simulink model "heyangjiang"  (Simulink 6.0)
settings: Solver=ode45  StartTime=0.0  StopTime=10.0  RelTol=1e-3
libraries: dsparch4 x2, commchan2 x1, dspxfrm3 x1, commsynccomp2 x1
settings Model: LastModifiedBy=xxgcxy602

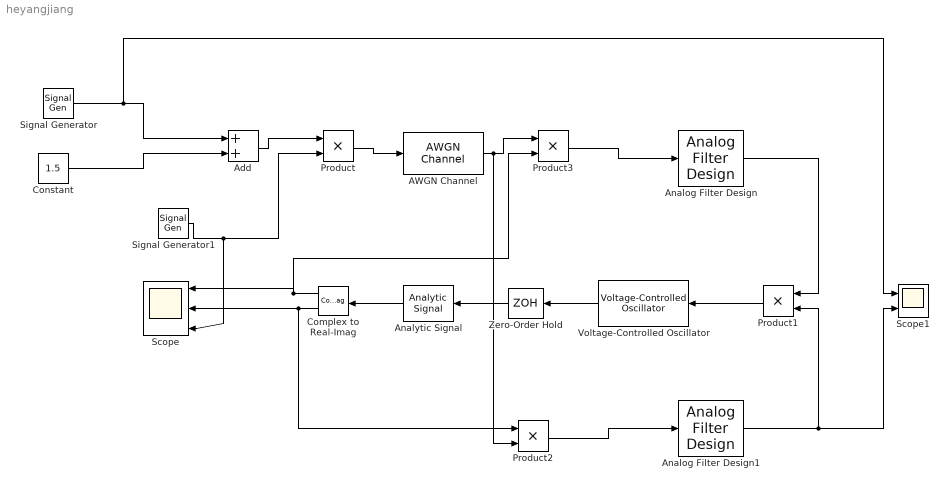
== system heyangjiang ==
  AWGN Channel : commchan2/AWGN Channel  seed=0  noiseMode=Variance from mask  EbNodB=10  EsNodB=10  SNRdB=10  bitsPerSym=1  Ps=1  Tsym=1  variance=0.01
  Add : Sum  OutScaling=2^-10
  Analog Filter Design : dsparch4/Analog Filter Design  method=Butterworth  filttype=Lowpass  N=1  Wlo=2000*2*pi  Whi=80  Rp=2  Rs=40
  Analog Filter Design1 : dsparch4/Analog Filter Design  method=Butterworth  filttype=Lowpass  N=8  Wlo=1000*2*pi  Whi=80  Rp=2  Rs=40
  Analytic Signal : dspxfrm3/Analytic Signal  Orientation=left  N=100
  Complex to Real-Imag : ComplexToRealImag  Orientation=left
  Constant : Constant  Value=1.5
  Product : Product  RndMeth=Zero
  Product1 : Product  Orientation=left  RndMeth=Zero
  Product2 : Product  RndMeth=Zero
  Product3 : Product  RndMeth=Zero
  Scope : Scope  NumInputPorts=3
      settings: YMin=-5~-5~-5  YMax=5~5~5
  Scope1 : Scope  NumInputPorts=2
      settings: YMin=-1~-1.25  YMax=1~-0.25
  Signal Generator : SignalGenerator  Frequency=1000
  Signal Generator1 : SignalGenerator  Amplitude=1.5  Frequency=10000
  Voltage-Controlled Oscillator : commsynccomp2/Voltage-Controlled Oscillator  Orientation=left  Ac=1  Fc=10150  Kc=1000  Ph=0
  Zero-Order Hold : ZeroOrderHold  Orientation=left  SampleTime=0.000001
  wires:
  Signal Generator/1 -> Add/1, Scope1/1
  Constant/1 -> Add/2
  Analog Filter Design/1 -> Product1/1
  Product1/1 -> Voltage-Controlled Oscillator/1
  Voltage-Controlled Oscillator/1 -> Zero-Order Hold/1
  Zero-Order Hold/1 -> Analytic Signal/1
  Analytic Signal/1 -> Complex to Real-Imag/1
  Complex to Real-Imag/1 -> Scope/1, Product3/2
  Complex to Real-Imag/2 -> Scope/2, Product2/1
  Signal Generator1/1 -> Product/2, Scope/3
  Add/1 -> Product/1
  Product/1 -> AWGN Channel/1
  AWGN Channel/1 -> Product3/1, Product2/2
  Product3/1 -> Analog Filter Design/1
  Product2/1 -> Analog Filter Design1/1
  Analog Filter Design1/1 -> Product1/2, Scope1/2
